simulink model "PID_Change"  (R2020b)
settings: Solver=VariableStepAuto  StartTime=0.0  StopTime=30  RelTol=1e-3
settings Model: Creator=Administrator  LastModifiedBy=Administrator

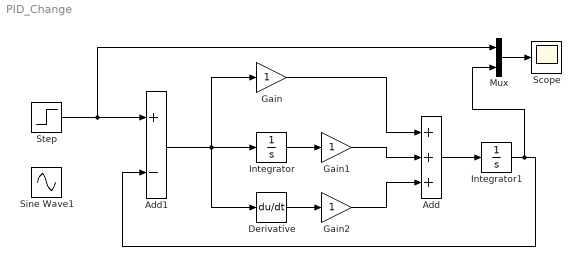
== system PID_Change ==
  Add : Sum  Inputs=+++
  Add1 : Sum  Inputs=+-
  Derivative : Derivative
  Gain : Gain
  Gain1 : Gain
  Gain2 : Gain
  Integrator : Integrator
  Integrator1 : Integrator
  Mux : Mux  Inputs=2
  Scope : Scope
  Sine Wave1 : Sin  SampleTime=0
  Step : Step  Time=0  SampleTime=0
  wires:
  Integrator/1 -> Gain1/1
  Derivative/1 -> Gain2/1
  Gain/1 -> Add/1
  Gain1/1 -> Add/2
  Gain2/1 -> Add/3
  Step/1 -> Mux/1, Add1/1
  Add/1 -> Integrator1/1
  Integrator1/1 -> Mux/2, Add1/2
  Add1/1 -> Derivative/1, Integrator/1, Gain/1
  Mux/1 -> Scope/1
